simulink model "three"  (R2020b)
settings: Solver=ode45  StartTime=0.0  StopTime=100  RelTol=1e-3  AbsTol=1e-6
values from neighbouring files (symbols this model uses):
  b1 = 350.0    [sus_para.sldd]
  b2 = 15020.0    [sus_para.sldd]
  k1 = 80000.0    [sus_para.sldd]
  k2 = 500000.0    [sus_para.sldd]
  m1 = 2500.0    [sus_para.sldd]
  m2 = 320.0    [sus_para.sldd]
settings Model: DataDictionary=sus_para.sldd  Creator=USER  LastModifiedBy=USER

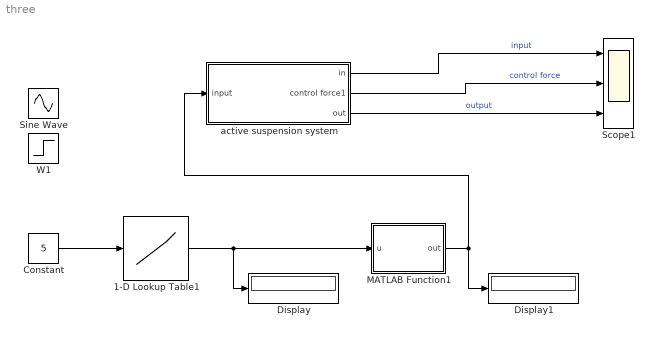
== system three ==
  1-D Lookup Table1 : Lookup_n-D  NumberOfTableDimensions=1  BreakpointsForDimension1=[0:10]  Table=[1,1.1,1.2,1.3,1.4,1.5,1.6,1.7,1.8,1.9,2]  InternalRulePriority=Speed  RndMeth=Simplest  InputSameDT=on
  Constant : Constant  Value=5
  Display : Display
  Display1 : Display
  MATLAB Function1 : MATLAB Function  TreatAsAtomicUnit=on
  Scope1 : Scope  NumInputPorts=3
  Sine Wave : Sin  SampleTime=0
  W1 : Step  Time=0  After=0
  active suspension system : Subsystem
  wires:
  active suspension system/1(in) -> Scope1/1  "input"
  active suspension system/2(control force1) -> Scope1/2  "control force"
  active suspension system/3(out) -> Scope1/3  "output"
  1-D Lookup Table1/1 -> MATLAB Function1/1(u), Display/1
  Constant/1 -> 1-D Lookup Table1/1
  MATLAB Function1/1(out) -> active suspension system/1(input), Display1/1

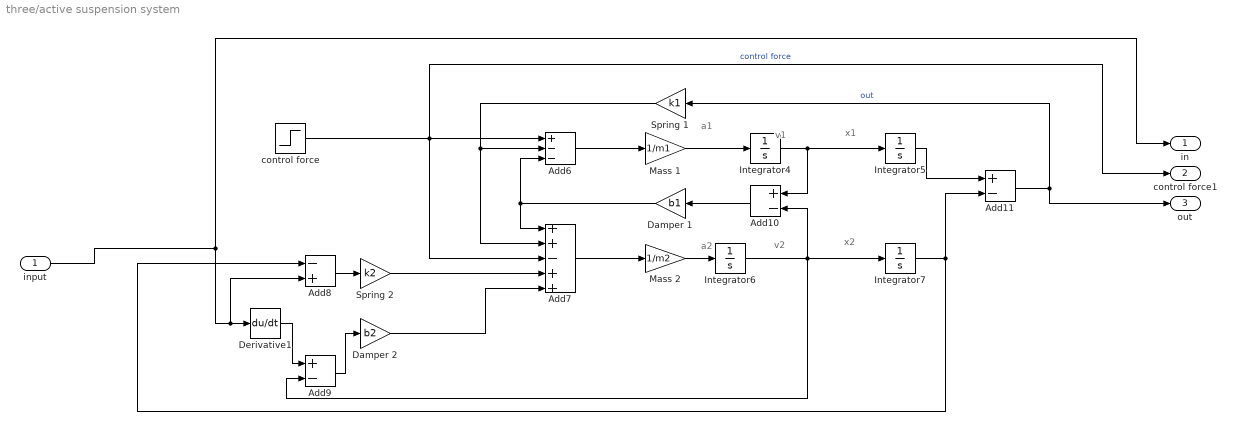
== system three/active suspension system ==
  note: v1
  note: a2
  note: v2
  note: x1
  note: a1
  note: x2
  input : Inport
  Add10 : Sum  Inputs=+-
  Add11 : Sum  Inputs=+-
  Add6 : Sum  Inputs=+--
  Add7 : Sum  Inputs=++-++
  Add8 : Sum  Inputs=-+
  Add9 : Sum  Inputs=+-
  Damper 1 : Gain  Gain=b1
  Damper 2 : Gain  Gain=b2
  Derivative1 : Derivative
  Integrator{4..7} (4 alike) : Integrator
  Mass 1 : Gain  Gain=1/m1
  Mass 2 : Gain  Gain=1/m2
  Spring 1 : Gain  Gain=k1
  Spring 2 : Gain  Gain=k2
  control force : Step  SampleTime=0
  in : Outport
  control force1 : Outport  Port=2
  out : Outport  Port=3
  wires:
  Integrator6/1 -> Add10/2, Integrator7/1, Add9/2
  control force/1 -> control force1/1, Add7/3, Add6/1  "control force"
  Spring 2/1 -> Add7/4
  Damper 2/1 -> Add7/5
  Add11/1 -> out/1, Spring 1/1  "out"
  input/1 -> in/1, Derivative1/1, Add8/2
  Damper 1/1 -> Add7/1, Add6/3
  Add8/1 -> Spring 2/1
  Integrator7/1 -> Add8/1, Add11/2
  Spring 1/1 -> Add7/2, Add6/2
  Add9/1 -> Damper 2/1
  Add7/1 -> Mass 2/1
  Integrator5/1 -> Add11/1
  Add6/1 -> Mass 1/1
  Mass 1/1 -> Integrator4/1
  Mass 2/1 -> Integrator6/1
  Integrator4/1 -> Add10/1, Integrator5/1
  Derivative1/1 -> Add9/1
  Add10/1 -> Damper 1/1

== matlab function three/MATLAB Function1 ==
  data: u input; out output
function out = fcn(u)
if(u>1.5)
    out=1;
else
    out=u;

end
